simulink model "AC_AC"  (R2021b)
settings: Solver=VariableStepAuto  StartTime=0.0  StopTime=1  RelTol=1e-3
libraries: spsSeriesRLCBranchLib x12, spsMosfetLib x8, spsRMSLib x5, spsCurrentMeasurementLib x4, slpidlib x3, spsMeanLib x2, simulink x2, spsVoltageMeasurementLib x2, spsACVoltageSourceLib x1, powerlib_extras x1, spsTHDLib x1, spspowerguiLib x1
settings Model: SimulationMode=accelerator  Creator=t'c  LastModifiedBy=abc6820292
settings SolverCC: AlgebraicLoopSolver=TrustRegion
settings DebuggingCC: UnconnectedInputMsg=none  UnconnectedOutputMsg=none  UnconnectedLineMsg=none  SFMachineParentedDataDiag=warning
settings ModelReferenceCC: EnableRefExpFcnMdlSchedulingChecks=off
settings SFSimCC: CustomCodeUndefinedFunction=UseInterfaceOnly

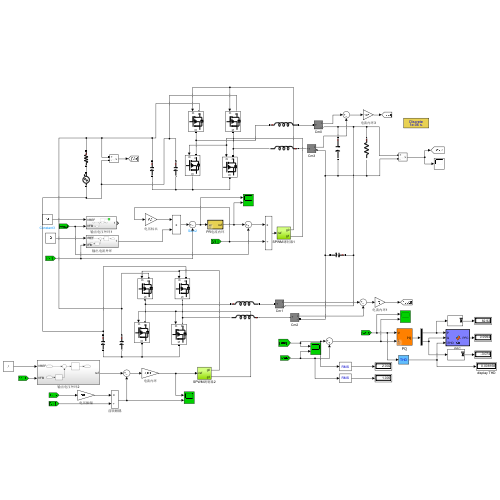
[thumbnail: Simulink's stored preview of the top-level diagram]
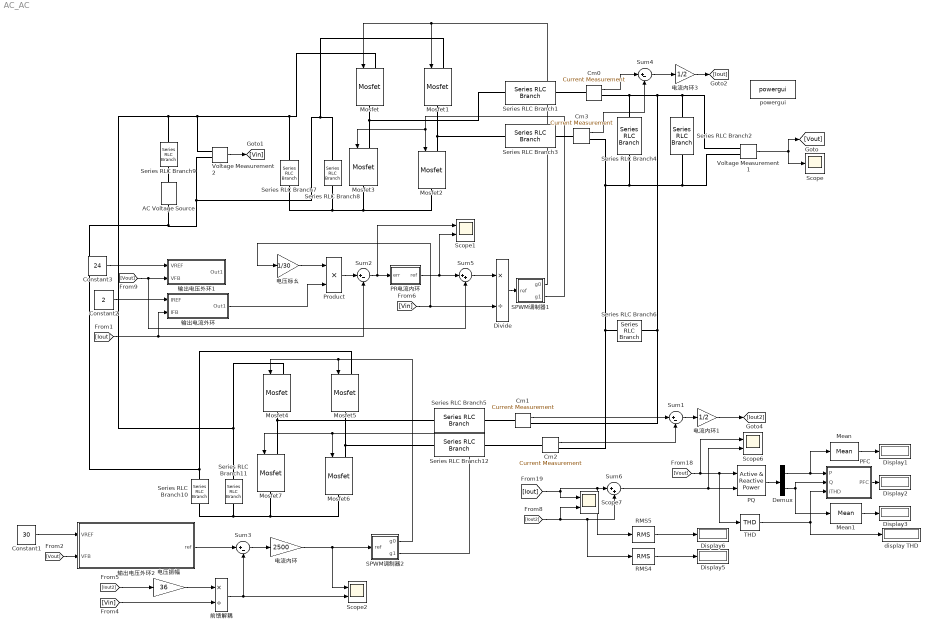
== system AC_AC ==
  AC Voltage Source : spsACVoltageSourceLib/AC Voltage Source  Amplitude=36*sqrt(2)  Phase=0  Frequency=50  SampleTime=0  Measurements=Voltage  BusType=swing  Pref=10e3  Qref=0  Qmin=-inf  Qmax=+inf
  Cm{0..3} (4 alike) : spsCurrentMeasurementLib/Current Measurement  PhasorSimulation=off  OutputType=Complex  PSBequivalent=0
  Constant1 : Constant  Value=30
  Constant2 : Constant  Value=2
  Constant3 : Constant  Value=24
  Demux : Demux  Outputs=2
  Display{1..3,5..6} (5 alike) : Display
  Divide : Product  Inputs=*/
  Mean : spsMeanLib/Mean  Freq=50  Vinit=0  Ts=0
  Mean1 : spsMeanLib/Mean  Freq=50  Vinit=0  Ts=0
  Mosfet{,1..7} (8 alike) : spsMosfetLib/Mosfet  Ron=0.01  Lon=0  Rd=0.01  Vfd=0  IC=0  Rs=1e5  Cs=inf  Measurements=off
  PFC : MATLAB Function  TreatAsAtomicUnit=on
  PQ : powerlib_extras/Measurements/Active & Reactive Power  f1=60
      settings: SourceProductBaseCode=PS
  PR电流内环 : Subsystem  TreatAsAtomicUnit=on  mask{Kp=4, Kr=100, Wc=5, Upper=200, Lower=-200}
  Product : Product
  RMS4 : spsRMSLib/RMS  TrueRMS=on  Freq=50  RMSInit=0  Ts=0
  RMS5 : spsRMSLib/RMS  TrueRMS=on  Freq=50  RMSInit=0  Ts=0
  SPWM调制器1 : Subsystem
  SPWM调制器2 : Subsystem
  Scope : Scope
  Scope{1..2,6..7} (4 alike) : Scope  NumInputPorts=2
  Series RLC Branch{1,3,5,12} (4 alike) : spsSeriesRLCBranchLib/Series RLC Branch  LConnTagsString=__new0  RConnTagsString=__new0  BranchType=L  Resistance=10  Inductance=3e-4  SetiL0=off  InitialCurrent=0  Capacitance=1e-6  Setx0=off  InitialVoltage=0  Measurements=Branch voltage
  Series RLC Branch{4,6..8,10..11} (6 alike) : spsSeriesRLCBranchLib/Series RLC Branch  LConnTagsString=__new0  RConnTagsString=__new0  BranchType=C  Resistance=10  Inductance=1e-3  SetiL0=off  InitialCurrent=0  Capacitance=6e-6  Setx0=off  InitialVoltage=0  Measurements=Branch voltage
  Series RLC Branch2 : spsSeriesRLCBranchLib/Series RLC Branch  LConnTagsString=__new0  RConnTagsString=__new0  BranchType=R  Resistance=10  Inductance=1e-3  SetiL0=off  InitialCurrent=0  Capacitance=1e-6  Setx0=off  InitialVoltage=0  Measurements=Branch voltage
  Series RLC Branch9 : spsSeriesRLCBranchLib/Series RLC Branch  LConnTagsString=__new0  RConnTagsString=__new0  BranchType=R  Resistance=0.01  Inductance=1e-3  SetiL0=off  InitialCurrent=0  Capacitance=6e-6  Setx0=off  InitialVoltage=0  Measurements=Branch voltage
  Sum{1..4} (4 alike) : Sum  Inputs=|+-
  Sum5 : Sum  Inputs=|++
  Sum6 : Sum  Inputs=|++
  THD : spsTHDLib/THD  Freq=50  Ts=0
      settings: SourceProductBaseCode=PS
  Voltage Measurement1 : spsVoltageMeasurementLib/Voltage Measurement  PhasorSimulation=off  OutputType=Complex  PSBequivalent=0
  Voltage Measurement2 : spsVoltageMeasurementLib/Voltage Measurement  PhasorSimulation=off  OutputType=Complex  PSBequivalent=0
  display THD : Display
  powergui : spspowerguiLib/powergui  SimulationMode=Discrete  SampleTime=1e-6  frequency=60  Iterations=50  frequencyindice=0  Pbase=100e6  ErrMax=1e-4  UnitsV=kV  UnitsW=MW  buscounter=0  FunctionMessages=off  echomessages=off  EnableUseOfTLC=off  CurrentSourceSwitches=off  DisableSnubberDevices=off  DisableRonSwitches=off  DisableVfSwitches=off  DisplayEquations=off  AutomaticDiscreteSolvers=off  SolverType=Tustin/Backward Euler (TBE)  Interpol=off  ExternalGateDelay=off  methode=off  Ts=0  x0status=blocks  SPID=off  SwTol=0  HookPort=off  NonlinearTolerance=1e-4  nMaxIteration=100  ContinueOnMaxIteration=off  RestoreLinks=warning  ResistiveCurrentMeasurement=off  Frange=[0:2:500]  Ylog=off  Xlog=on  ShowGrid=off  save=off  variable=ZData  structure=QQQQQ  ZoomFFT=off  StartTime=0.5  cycles=15  DisplayStyle=1  fundamental=50  FreqAxis=off  MaxFrequency=1000  frequencyindicesteady=1  RmsSteady=1  display=off
  前馈解耦 : Product  Inputs=*/
  电压振幅 : Gain  Gain=36
  电压标幺 : Gain  Gain=1/30
  电流内环 : Gain  Gain=2500
  电流内环1 : Gain  Gain=1/2
  电流内环3 : Gain  Gain=1/2
  输出电压外环1 : Subsystem
  输出电压外环2 : Subsystem
  输出电流外环 : Subsystem
  wires:
  Voltage Measurement1/1 -> Scope/1, [Vout]
  Demux/1 -> Mean/1, PFC/1(P)
  PQ/1 -> Demux/1
  Mean1/1 -> Display3/1
  Mean/1 -> Display1/1
  PFC/1(PFC) -> Display2/1
  [Vout] -> Scope6/1, THD/1, PQ/1
  THD/1 -> PFC/3(iTHD), display THD/1
  Demux/2 -> PFC/2(Q), Mean1/1
  Voltage Measurement2/1 -> [Vin]
  [Iout] -> Sum2/2, 输出电流外环/2(IFB)
  [Iout] -> Scope7/1, RMS5/1, Sum6/1
  [Iout2] -> Scope7/2, RMS4/1, Sum6/2
  Sum6/1 -> Scope6/2, PQ/2
  RMS4/1 -> Display5/1
  RMS5/1 -> Display6/1
  Constant1/1 -> 输出电压外环2/1(VREF)
  [Vin] -> 前馈解耦/2
  Constant3/1 -> 输出电压外环1/1(VREF)
  Constant2/1 -> 输出电流外环/1(IREF)
  [Vout] -> 输出电压外环2/2(VFB)
  [Vout] -> 输出电压外环1/2(VFB), Sum5/2
  输出电压外环2/1(ref) -> Sum3/1
  前馈解耦/1 -> Sum3/2, Scope2/2
  Sum3/1 -> 电流内环/1
  电流内环/1 -> Scope2/1, SPWM调制器2/1(ref)
  [Vin] -> 电压标幺/1, Divide/2
  Divide/1 -> SPWM调制器1/1(ref)
  PR电流内环/1(ref) -> Scope1/2, Sum5/1
  Sum2/1 -> Scope1/1, PR电流内环/1(err)
  Product/1 -> Sum2/1
  电压标幺/1 -> Product/1
  SPWM调制器1/1(g0) -> Mosfet/1, Mosfet1/1
  SPWM调制器1/2(g1) -> Mosfet3/1, Mosfet2/1
  SPWM调制器2/2(g1) -> Mosfet7/1, Mosfet6/1
  SPWM调制器2/1(g0) -> Mosfet4/1, Mosfet5/1
  输出电流外环/1(Out1) -> Product/2
  Cm1/1 -> Sum1/1
  Cm2/1 -> Sum1/2
  Sum1/1 -> 电流内环1/1
  电流内环1/1 -> [Iout2]
  Cm0/1 -> Sum4/1
  Cm3/1 -> Sum4/2
  Sum4/1 -> 电流内环3/1
  电流内环3/1 -> [Iout]
  Sum5/1 -> Divide/1
  [Iout2] -> 电压振幅/1
  电压振幅/1 -> 前馈解耦/1
  connections:
  Voltage Measurement2/LConn2 -- Series RLC Branch8/LConn1 -- Mosfet1/LConn1 -- Mosfet5/LConn1 -- Series RLC Branch10/LConn1 -- AC Voltage Source/LConn1
  Voltage Measurement2/LConn1 -- Series RLC Branch7/LConn1 -- Mosfet/LConn1 -- Mosfet4/LConn1 -- Series RLC Branch11/LConn1 -- Series RLC Branch9/LConn1
  Series RLC Branch5/RConn1 -- Cm1/LConn1
  Mosfet/RConn1 -- Mosfet3/LConn1 -- Series RLC Branch1/LConn1
  Mosfet2/LConn1 -- Series RLC Branch3/RConn1 -- Mosfet1/RConn1
  Series RLC Branch7/RConn1 -- Series RLC Branch8/RConn1 -- Mosfet2/RConn1 -- Mosfet3/RConn1
  Series RLC Branch9/RConn1 -- AC Voltage Source/RConn1
  Mosfet7/RConn1 -- Series RLC Branch11/RConn1 -- Series RLC Branch10/RConn1 -- Mosfet6/RConn1
  Mosfet6/LConn1 -- Mosfet5/RConn1 -- Series RLC Branch12/RConn1
  Mosfet4/RConn1 -- Mosfet7/LConn1 -- Series RLC Branch5/LConn1
  Series RLC Branch1/RConn1 -- Cm0/LConn1
  Cm0/RConn1 -- Cm1/RConn1 -- Series RLC Branch6/LConn1 -- Voltage Measurement1/LConn1 -- Series RLC Branch2/LConn1 -- Series RLC Branch4/LConn1
  Series RLC Branch4/RConn1 -- Series RLC Branch6/RConn1 -- Cm2/RConn1 -- Cm3/RConn1 -- Voltage Measurement1/LConn2 -- Series RLC Branch2/RConn1
  Cm2/LConn1 -- Series RLC Branch12/LConn1
  Cm3/LConn1 -- Series RLC Branch3/LConn1

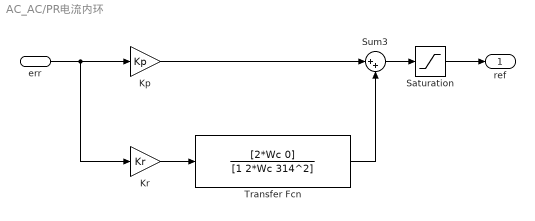
== system AC_AC/PR电流内环 ==
  err : Inport
  Kp : Gain  Gain=Kp
  Kr : Gain  Gain=Kr
  Saturation : Saturate  UpperLimit=Upper  LowerLimit=Lower
  Sum3 : Sum  Inputs=|++
  Transfer Fcn : TransferFcn  Numerator=[2*Wc 0]  Denominator=[1 2*Wc 314^2]
  ref : Outport
  wires:
  Kp/1 -> Sum3/1
  Sum3/1 -> Saturation/1
  err/1 -> Kr/1, Kp/1
  Kr/1 -> Transfer Fcn/1
  Transfer Fcn/1 -> Sum3/2
  Saturation/1 -> ref/1

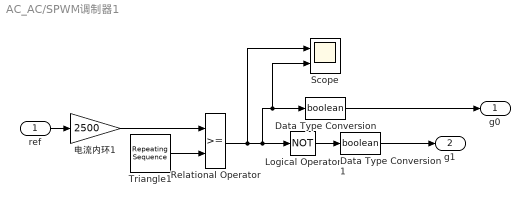
== system AC_AC/SPWM调制器1 ==
  ref : Inport
  Data Type Conversion : DataTypeConversion  OutDataTypeStr=boolean
  Data Type Conversion1 : DataTypeConversion  OutDataTypeStr=boolean
  Logical Operator : Logic  Operator=NOT  AllPortsSameDT=off  OutDataTypeStr=boolean
  Relational Operator : RelationalOperator  OutDataTypeStr=boolean  RndMeth=Nearest
  Scope : Scope  NumInputPorts=2
  Triangle1 : simulink/Sources/Repeating Sequence  rep_seq_t=[0 1/30000/2 1/30000]  rep_seq_y=[0 2500 0]
  电流内环1 : Gain  Gain=2500
  g0 : Outport
  g1 : Outport  Port=2
  wires:
  Data Type Conversion/1 -> g0/1
  Logical Operator/1 -> Data Type Conversion1/1
  Data Type Conversion1/1 -> g1/1
  Relational Operator/1 -> Scope/1, Logical Operator/1, Scope/2, Data Type Conversion/1
  Triangle1/1 -> Relational Operator/2
  ref/1 -> 电流内环1/1
  电流内环1/1 -> Relational Operator/1

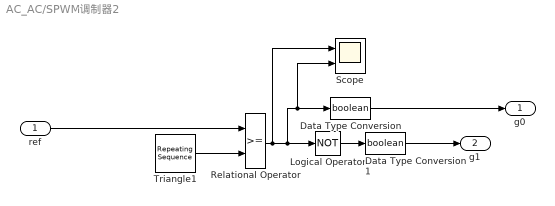
== system AC_AC/SPWM调制器2 ==
  ref : Inport
  Data Type Conversion : DataTypeConversion  OutDataTypeStr=boolean
  Data Type Conversion1 : DataTypeConversion  OutDataTypeStr=boolean
  Logical Operator : Logic  Operator=NOT  AllPortsSameDT=off  OutDataTypeStr=boolean
  Relational Operator : RelationalOperator  OutDataTypeStr=boolean  RndMeth=Nearest
  Scope : Scope  NumInputPorts=2
  Triangle1 : simulink/Sources/Repeating Sequence  rep_seq_t=[0 1/30000/2 1/30000]  rep_seq_y=[0 2500 0]
  g0 : Outport
  g1 : Outport  Port=2
  wires:
  Data Type Conversion/1 -> g0/1
  Logical Operator/1 -> Data Type Conversion1/1
  Data Type Conversion1/1 -> g1/1
  Relational Operator/1 -> Scope/1, Logical Operator/1, Scope/2, Data Type Conversion/1
  Triangle1/1 -> Relational Operator/2
  ref/1 -> Relational Operator/1

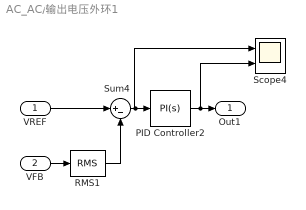
== system AC_AC/输出电压外环1 ==
  VREF : Inport
  VFB : Inport  Port=2
  PID Controller2 : slpidlib/PID Controller  Controller=PI  Form=Parallel  TimeDomain=Continuous-time  UseExternalTs=off  SampleTime=-1  IntegratorMethod=Forward Euler  FilterMethod=Forward Euler  ControllerParametersSource=internal  P=0.02  I=1  D=0  UseFilter=on  N=100  TunerSelectOption=Transfer Function Based (PID Tuner App)  InitialConditionSource=internal  InitialConditionForIntegrator=0  InitialConditionForFilter=0  DifferentiatorICPrevScaledInput=0  ExternalReset=none  TrackingMode=off  Kt=1  LimitOutput=on  SatLimitsSource=internal  UpperSaturationLimit=50  LowerSaturationLimit=0  LinearizeAsGain=on  AntiWindupMode=none  Kb=1  POutMin=[]  POutMax=[]  IOutMin=[]  IOutMax=[]  DOutMin=[]  DOutMax=[]  NOutMin=[]  NOutMax=[]  SumOutMin=[]  SumOutMax=[]  SaturationOutMin=[]  SaturationOutMax=[]  PParamMin=[]  PParamMax=[]  IParamMin=[]  IParamMax=[]  DParamMin=[]  DParamMax=[]  NParamMin=[]  NParamMax=[]  KbParamMin=[]  KbParamMax=[]  KtParamMin=[]  KtParamMax=[]  KbOutMin=[]  KbOutMax=[]  KtOutMin=[]  KtOutMax=[]  IntegratorOutMin=[]  IntegratorOutMax=[]  FilterOutMin=[]  FilterOutMax=[]  SumI1OutMin=[]  SumI1OutMax=[]  SumI2OutMin=[]  SumI2OutMax=[]  SumI3OutMin=[]  SumI3OutMax=[]  SumI4OutMin=[]  SumI4OutMax=[]  SumDOutMin=[]  SumDOutMax=[]  DifferentiatorOutMin=[]  DifferentiatorOutMax=[]  FilterDiffOutCoefMin=[]  FilterDiffOutCoefMax=[]  ReciprocalOutMin=[]  ReciprocalOutMax=[]  SumDenOutMin=[]  SumDenOutMax=[]  SumNumOutMin=[]  SumNumOutMax=[]  DivideOutMin=[]  DivideOutMax=[]  UdiffTsProdOutMin=[]  UdiffTsProdOutMax=[]  NTsProdOutMin=[]  NTsProdOutMax=[]  UintegralTsProdOutMin=[]  UintegralTsProdOutMax=[]  UngainTsProdOutMin=[]  UngainTsProdOutMax=[]  FilterDenConstantOutDataTypeStr=Inherit: Inherit via back propagation  FilterDenConstantOutMin=[]  FilterDenConstantOutMax=[]  PCopyOutDataTypeStr=Inherit: Inherit via back propagation  PCopyOutMin=[]  PCopyOutMax=[]  NCopyOutDataTypeStr=Inherit: Inherit via back propagation  NCopyOutMin=[]  NCopyOutMax=[]  IntegratorContinuousStateAttributes=''  IntegratorStateMustResolveToSignalObject=off  IntegratorRTWStateStorageClass=Auto  FilterContinuousStateAttributes=''  FilterStateMustResolveToSignalObject=off  FilterRTWStateStorageClass=Auto  ParallelPVariant=InternalParameters  IdealPVariant=Disabled  IVariant=InternalParameters  DVariant=Disabled  IntegratorVariant=Continuous  SatVariant=Enabled  AWVariant=Passthrough  PCopyVariant=Disabled  TRVariant=Disabled  FdbkBlocksVariant=Forward  IdealPFdbkVariant=Disabled  SatFdbkVariant=Disabled  DerivativeFilterVariant=Disabled  NVariant=Disabled  NCopyVariant=Disabled_SignalSpec  FilterICVariant=Disabled  IntegratorICVariant=InternalICs  ExternalResetVariant=Disabled  TRSumVariant=Passthrough  SumFdbkVariant=Disabled  SumVariant=Sum_PI  TsampFilterVariant=InternalTs  TsampNgainVariant=Passthrough  TsampIntegralVariant=Passthrough  ExternalSaturationOutDataTypeStr=Inherit: Same as second input
  RMS1 : spsRMSLib/RMS  TrueRMS=on  Freq=50  RMSInit=0  Ts=0
  Scope4 : Scope  NumInputPorts=2
  Sum4 : Sum  Inputs=|+-
  Out1 : Outport
  wires:
  VFB/1 -> RMS1/1
  RMS1/1 -> Sum4/2
  VREF/1 -> Sum4/1
  Sum4/1 -> Scope4/1, PID Controller2/1
  PID Controller2/1 -> Scope4/2, Out1/1

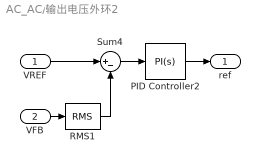
== system AC_AC/输出电压外环2 ==
  VREF : Inport
  VFB : Inport  Port=2
  PID Controller2 : slpidlib/PID Controller  Controller=PI  Form=Parallel  TimeDomain=Continuous-time  UseExternalTs=off  SampleTime=-1  IntegratorMethod=Forward Euler  FilterMethod=Forward Euler  ControllerParametersSource=internal  P=0.02  I=1  D=0  UseFilter=on  N=100  TunerSelectOption=Transfer Function Based (PID Tuner App)  InitialConditionSource=internal  InitialConditionForIntegrator=0  InitialConditionForFilter=0  DifferentiatorICPrevScaledInput=0  ExternalReset=none  TrackingMode=off  Kt=1  LimitOutput=on  SatLimitsSource=internal  UpperSaturationLimit=10  LowerSaturationLimit=0  LinearizeAsGain=on  AntiWindupMode=none  Kb=1  POutMin=[]  POutMax=[]  IOutMin=[]  IOutMax=[]  DOutMin=[]  DOutMax=[]  NOutMin=[]  NOutMax=[]  SumOutMin=[]  SumOutMax=[]  SaturationOutMin=[]  SaturationOutMax=[]  PParamMin=[]  PParamMax=[]  IParamMin=[]  IParamMax=[]  DParamMin=[]  DParamMax=[]  NParamMin=[]  NParamMax=[]  KbParamMin=[]  KbParamMax=[]  KtParamMin=[]  KtParamMax=[]  KbOutMin=[]  KbOutMax=[]  KtOutMin=[]  KtOutMax=[]  IntegratorOutMin=[]  IntegratorOutMax=[]  FilterOutMin=[]  FilterOutMax=[]  SumI1OutMin=[]  SumI1OutMax=[]  SumI2OutMin=[]  SumI2OutMax=[]  SumI3OutMin=[]  SumI3OutMax=[]  SumI4OutMin=[]  SumI4OutMax=[]  SumDOutMin=[]  SumDOutMax=[]  DifferentiatorOutMin=[]  DifferentiatorOutMax=[]  FilterDiffOutCoefMin=[]  FilterDiffOutCoefMax=[]  ReciprocalOutMin=[]  ReciprocalOutMax=[]  SumDenOutMin=[]  SumDenOutMax=[]  SumNumOutMin=[]  SumNumOutMax=[]  DivideOutMin=[]  DivideOutMax=[]  UdiffTsProdOutMin=[]  UdiffTsProdOutMax=[]  NTsProdOutMin=[]  NTsProdOutMax=[]  UintegralTsProdOutMin=[]  UintegralTsProdOutMax=[]  UngainTsProdOutMin=[]  UngainTsProdOutMax=[]  FilterDenConstantOutDataTypeStr=Inherit: Inherit via back propagation  FilterDenConstantOutMin=[]  FilterDenConstantOutMax=[]  PCopyOutDataTypeStr=Inherit: Inherit via back propagation  PCopyOutMin=[]  PCopyOutMax=[]  NCopyOutDataTypeStr=Inherit: Inherit via back propagation  NCopyOutMin=[]  NCopyOutMax=[]  IntegratorContinuousStateAttributes=''  IntegratorStateMustResolveToSignalObject=off  IntegratorRTWStateStorageClass=Auto  FilterContinuousStateAttributes=''  FilterStateMustResolveToSignalObject=off  FilterRTWStateStorageClass=Auto  ParallelPVariant=InternalParameters  IdealPVariant=Disabled  IVariant=InternalParameters  DVariant=Disabled  IntegratorVariant=Continuous  SatVariant=Enabled  AWVariant=Passthrough  PCopyVariant=Disabled  TRVariant=Disabled  FdbkBlocksVariant=Forward  IdealPFdbkVariant=Disabled  SatFdbkVariant=Disabled  DerivativeFilterVariant=Disabled  NVariant=Disabled  NCopyVariant=Disabled_SignalSpec  FilterICVariant=Disabled  IntegratorICVariant=InternalICs  ExternalResetVariant=Disabled  TRSumVariant=Passthrough  SumFdbkVariant=Disabled  SumVariant=Sum_PI  TsampFilterVariant=InternalTs  TsampNgainVariant=Passthrough  TsampIntegralVariant=Passthrough  ExternalSaturationOutDataTypeStr=Inherit: Same as second input
  RMS1 : spsRMSLib/RMS  TrueRMS=on  Freq=50  RMSInit=0  Ts=0
  Sum4 : Sum  Inputs=|+-
  ref : Outport
  wires:
  RMS1/1 -> Sum4/2
  VREF/1 -> Sum4/1
  PID Controller2/1 -> ref/1
  Sum4/1 -> PID Controller2/1
  VFB/1 -> RMS1/1

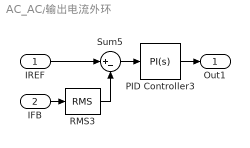
== system AC_AC/输出电流外环 ==
  IREF : Inport
  IFB : Inport  Port=2
  PID Controller3 : slpidlib/PID Controller  Controller=PI  Form=Parallel  TimeDomain=Continuous-time  UseExternalTs=off  SampleTime=-1  IntegratorMethod=Forward Euler  FilterMethod=Forward Euler  ControllerParametersSource=internal  P=0.01  I=10  D=0  UseFilter=on  N=100  TunerSelectOption=Transfer Function Based (PID Tuner App)  InitialConditionSource=internal  InitialConditionForIntegrator=0  InitialConditionForFilter=0  DifferentiatorICPrevScaledInput=0  ExternalReset=none  TrackingMode=off  Kt=1  LimitOutput=off  SatLimitsSource=internal  UpperSaturationLimit=10  LowerSaturationLimit=0  LinearizeAsGain=on  AntiWindupMode=none  Kb=1  POutMin=[]  POutMax=[]  IOutMin=[]  IOutMax=[]  DOutMin=[]  DOutMax=[]  NOutMin=[]  NOutMax=[]  SumOutMin=[]  SumOutMax=[]  SaturationOutMin=[]  SaturationOutMax=[]  PParamMin=[]  PParamMax=[]  IParamMin=[]  IParamMax=[]  DParamMin=[]  DParamMax=[]  NParamMin=[]  NParamMax=[]  KbParamMin=[]  KbParamMax=[]  KtParamMin=[]  KtParamMax=[]  KbOutMin=[]  KbOutMax=[]  KtOutMin=[]  KtOutMax=[]  IntegratorOutMin=[]  IntegratorOutMax=[]  FilterOutMin=[]  FilterOutMax=[]  SumI1OutMin=[]  SumI1OutMax=[]  SumI2OutMin=[]  SumI2OutMax=[]  SumI3OutMin=[]  SumI3OutMax=[]  SumI4OutMin=[]  SumI4OutMax=[]  SumDOutMin=[]  SumDOutMax=[]  DifferentiatorOutMin=[]  DifferentiatorOutMax=[]  FilterDiffOutCoefMin=[]  FilterDiffOutCoefMax=[]  ReciprocalOutMin=[]  ReciprocalOutMax=[]  SumDenOutMin=[]  SumDenOutMax=[]  SumNumOutMin=[]  SumNumOutMax=[]  DivideOutMin=[]  DivideOutMax=[]  UdiffTsProdOutMin=[]  UdiffTsProdOutMax=[]  NTsProdOutMin=[]  NTsProdOutMax=[]  UintegralTsProdOutMin=[]  UintegralTsProdOutMax=[]  UngainTsProdOutMin=[]  UngainTsProdOutMax=[]  FilterDenConstantOutDataTypeStr=Inherit: Inherit via back propagation  FilterDenConstantOutMin=[]  FilterDenConstantOutMax=[]  PCopyOutDataTypeStr=Inherit: Inherit via back propagation  PCopyOutMin=[]  PCopyOutMax=[]  NCopyOutDataTypeStr=Inherit: Inherit via back propagation  NCopyOutMin=[]  NCopyOutMax=[]  IntegratorContinuousStateAttributes=''  IntegratorStateMustResolveToSignalObject=off  IntegratorRTWStateStorageClass=Auto  FilterContinuousStateAttributes=''  FilterStateMustResolveToSignalObject=off  FilterRTWStateStorageClass=Auto  ParallelPVariant=InternalParameters  IdealPVariant=Disabled  IVariant=InternalParameters  DVariant=Disabled  IntegratorVariant=Continuous  SatVariant=Disabled  AWVariant=Passthrough  PCopyVariant=Disabled  TRVariant=Disabled  FdbkBlocksVariant=Forward  IdealPFdbkVariant=Disabled  SatFdbkVariant=Disabled  DerivativeFilterVariant=Disabled  NVariant=Disabled  NCopyVariant=Disabled_SignalSpec  FilterICVariant=Disabled  IntegratorICVariant=InternalICs  ExternalResetVariant=Disabled  TRSumVariant=Passthrough  SumFdbkVariant=Disabled  SumVariant=Sum_PI  TsampFilterVariant=InternalTs  TsampNgainVariant=Passthrough  TsampIntegralVariant=Passthrough  ExternalSaturationOutDataTypeStr=Inherit: Same as second input
  RMS3 : spsRMSLib/RMS  TrueRMS=on  Freq=50  RMSInit=0  Ts=0
  Sum5 : Sum  Inputs=|+-
  Out1 : Outport
  wires:
  IREF/1 -> Sum5/1
  RMS3/1 -> Sum5/2
  Sum5/1 -> PID Controller3/1
  PID Controller3/1 -> Out1/1
  IFB/1 -> RMS3/1

== matlab function AC_AC/PFC ==
  data: P input; PFC output; Q input; iTHD input
function PFC = fcn(P,Q,iTHD)
% This block supports an embeddable subset of the MATLAB language.
% See the help menu for details. 
PFC=(P/sqrt(P*P+Q*Q))/sqrt(1+iTHD^2);
